simulink model "encoder_M_T"  (R2012b)
settings: Solver=ode45  StartTime=0.0  StopTime=10.0  RelTol=1e-3
libraries: simulink x4
settings Model: Creator=Juliano  LastModifiedBy=Juliano

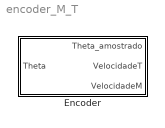
== system encoder_M_T ==
  Encoder : Subsystem  mask{Nr=500}
      mask prompts: Nr "Número de pulsos por revolução"

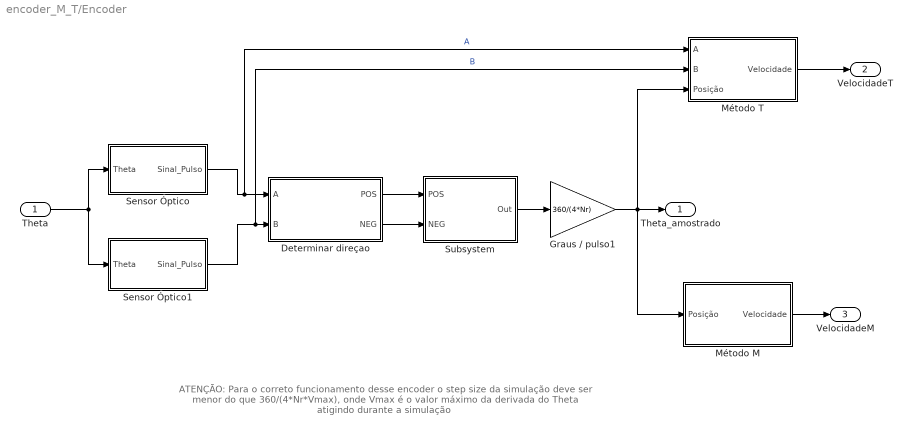
== system encoder_M_T/Encoder ==
  note: ATENÇÃO: Para o correto funcionamento desse encoder o step size da simulação deve ser menor do que 360/(4*Nr*Vmax),
      | onde Vmax é o valor máximo da derivada do Theta atigindo durante a simulação
  Theta : Inport
  Determinar direçao : Subsystem
  Graus / pulso1 : Gain  Gain=360/(4*Nr)  OutDataTypeStr=double
  Método M : Subsystem  mask{Ts=0.1}
      mask prompts: Ts "Sampling time"
  Método T : Subsystem  mask{m=10}
      mask prompts: m "Número de pulsos que o bloco espera para calcular a velocidade média"
  Sensor Óptico : Subsystem
  Sensor Óptico1 : Subsystem
  Subsystem : Subsystem
  Theta_amostrado : Outport
  VelocidadeT : Outport  Port=2
  VelocidadeM : Outport  Port=3
  wires:
  Método M/1(Velocidade) -> VelocidadeM/1
  Método T/1(Velocidade) -> VelocidadeT/1
  Theta/1 -> Sensor Óptico/1(Theta), Sensor Óptico1/1(Theta)
  Graus / pulso1/1 -> Theta_amostrado/1, Método T/3(Posição), Método M/1(Posição)
  Subsystem/1(Out) -> Graus / pulso1/1
  Determinar direçao/2(NEG) -> Subsystem/2(NEG)
  Determinar direçao/1(POS) -> Subsystem/1(POS)
  Sensor Óptico1/1(Sinal_Pulso) -> Determinar direçao/2(B), Método T/2(B)  "B"
  Sensor Óptico/1(Sinal_Pulso) -> Método T/1(A), Determinar direçao/1(A)  "A"

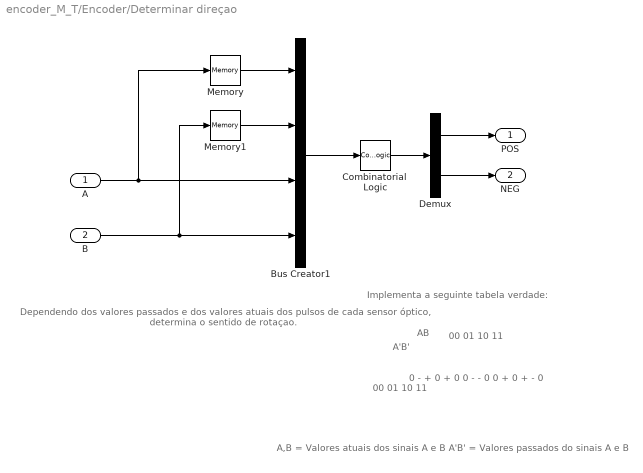
== system encoder_M_T/Encoder/Determinar direçao ==
  note: Dependendo dos valores passados e dos valores atuais
      | dos pulsos de cada sensor óptico, determina o sentido
      | de rotaçao.
  note: 00
      | 01
      | 10
      | 11
  note: 00 01 10 11
  note: 0	-	+	0
      | +	0	0	-
      | -	0	0	+
      | 0	+	-	0
  note: Implementa a seguinte tabela verdade:
  note: AB
  note: A'B'
  note: A,B = Valores atuais dos sinais A e B
      | A'B' = Valores passados do sinais A e B
  A : Inport
  B : Inport  Port=2
  Bus Creator1 : BusCreator
  Combinatorial  Logic : CombinatorialLogic  TruthTable=[ 0 0 ; 0 1 ; 1 0 ; 0 0 ; 1 0 ; 0 0 ; 0 0 ; 0 1 ; 0 1 ; 0 0 ; 0 0 ; 1 0 ; 0 0 ; 1 0 ; 0 1 ; 0 0]
  Demux : Demux  Outputs=2
  Memory : Memory
  Memory1 : Memory
  POS : Outport
  NEG : Outport  Port=2
  wires:
  B/1 -> Bus Creator1/4, Memory1/1
  Memory1/1 -> Bus Creator1/2
  Bus Creator1/1 -> Combinatorial  Logic/1
  Memory/1 -> Bus Creator1/1
  Combinatorial  Logic/1 -> Demux/1
  Demux/2 -> NEG/1
  A/1 -> Bus Creator1/3, Memory/1
  Demux/1 -> POS/1

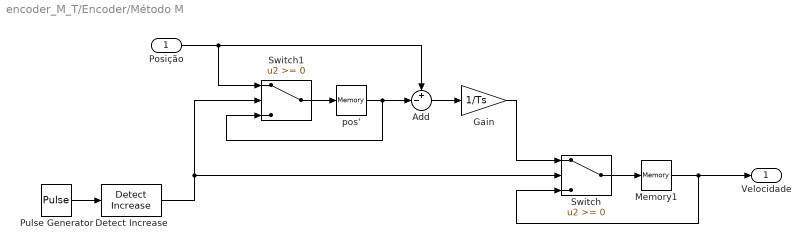
== system encoder_M_T/Encoder/Método M ==
  Posição : Inport
  Add : Sum  Inputs=+-|
  Detect Increase : simulink/Logic and Bit Operations/Detect Increase  vinit=0.0  InputProcessing=Inherited  OutDataTypeStr=boolean
  Gain : Gain  Gain=1/Ts
  Memory1 : Memory
  Pulse Generator : DiscretePulseGenerator  PulseType=Time based  Period=Ts  PulseWidth=50
  Switch : Switch
  Switch1 : Switch
  pos' : Memory
  Velocidade : Outport
  wires:
  Detect Increase/1 -> Switch1/2, Switch/2
  Gain/1 -> Switch/1
  Posição/1 -> Add/1, Switch1/1
  Memory1/1 -> Switch/3, Velocidade/1
  Switch/1 -> Memory1/1
  Switch1/1 -> pos'/1
  Add/1 -> Gain/1
  Pulse Generator/1 -> Detect Increase/1
  pos'/1 -> Switch1/3, Add/2

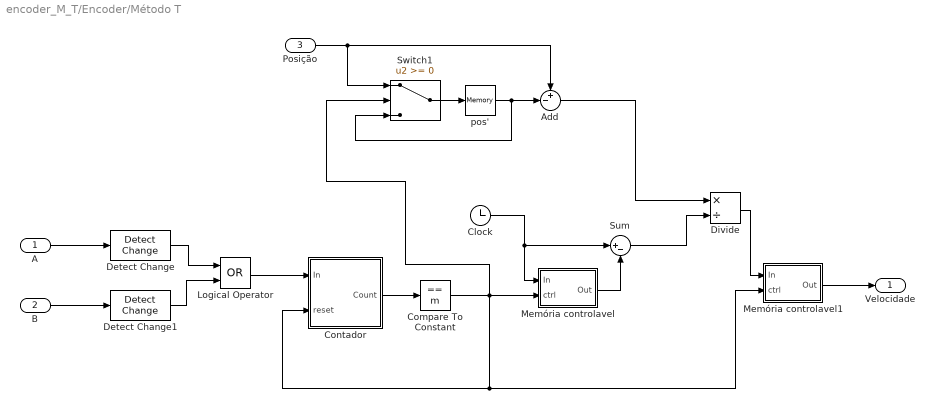
== system encoder_M_T/Encoder/Método T ==
  A : Inport
  B : Inport  Port=2
  Posição : Inport  Port=3
  Add : Sum  Inputs=+-|
  Clock : Clock
  Compare To Constant : simulink/Logic and Bit Operations/Compare To Constant  relop===  const=m  OutDataTypeStr=boolean
  Contador : Subsystem
  Detect Change : simulink/Logic and Bit Operations/Detect Change  vinit=0  InputProcessing=Inherited  OutDataTypeStr=boolean
  Detect Change1 : simulink/Logic and Bit Operations/Detect Change  vinit=0  InputProcessing=Inherited  OutDataTypeStr=boolean
  Divide : Product  Inputs=*/
  Logical Operator : Logic  Operator=OR  AllPortsSameDT=off  OutDataTypeStr=boolean
  Memória controlavel : Subsystem
  Memória controlavel1 : Subsystem
  Sum : Sum  Inputs=|+-
  Switch1 : Switch
  pos' : Memory
  Velocidade : Outport
  wires:
  Posição/1 -> Add/1, Switch1/1
  Switch1/1 -> pos'/1
  pos'/1 -> Switch1/3, Add/2
  Memória controlavel1/1(Out) -> Velocidade/1
  Compare To Constant/1 -> Memória controlavel/2(ctrl), Switch1/2, Contador/2(reset), Memória controlavel1/2(ctrl)
  Clock/1 -> Memória controlavel/1(In), Sum/1
  Add/1 -> Divide/1
  Sum/1 -> Divide/2
  Memória controlavel/1(Out) -> Sum/2
  Divide/1 -> Memória controlavel1/1(In)
  Contador/1(Count) -> Compare To Constant/1
  Logical Operator/1 -> Contador/1(In)
  Detect Change1/1 -> Logical Operator/2
  Detect Change/1 -> Logical Operator/1
  B/1 -> Detect Change1/1
  A/1 -> Detect Change/1

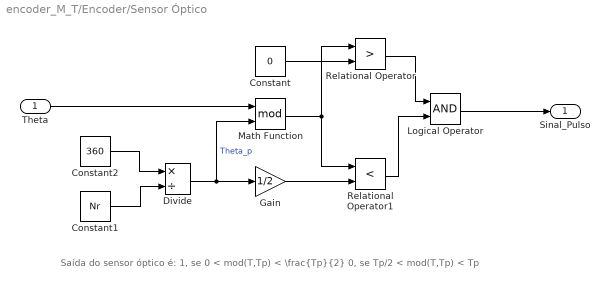
== system encoder_M_T/Encoder/Sensor Óptico ==
  note: Saída do sensor óptico é:
      | 1, se	0 < mod(T,Tp) < \frac{Tp}{2}
      |  0, se      Tp/2 < mod(T,Tp) < Tp
  Theta : Inport
  Constant : Constant  Value=0
  Constant1 : Constant  Value=Nr
  Constant2 : Constant  Value=360
  Divide : Product  Inputs=*/
  Gain : Gain  Gain=1/2
  Logical Operator : Logic  AllPortsSameDT=off  OutDataTypeStr=boolean
  Math Function : Math  Operator=mod  SaturateOnIntegerOverflow=on
  Relational Operator : RelationalOperator  Operator=>  OutDataTypeStr=boolean
  Relational Operator1 : RelationalOperator  Operator=<  OutDataTypeStr=boolean
  Sinal_Pulso : Outport
  wires:
  Constant1/1 -> Divide/2
  Constant2/1 -> Divide/1
  Logical Operator/1 -> Sinal_Pulso/1
  Gain/1 -> Relational Operator1/2
  Divide/1 -> Gain/1, Math Function/2  "Theta_p"
  Constant/1 -> Relational Operator/2
  Relational Operator1/1 -> Logical Operator/2
  Relational Operator/1 -> Logical Operator/1
  Theta/1 -> Math Function/1
  Math Function/1 -> Relational Operator/1, Relational Operator1/1

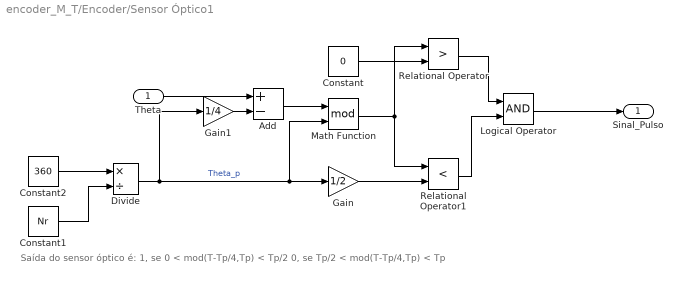
== system encoder_M_T/Encoder/Sensor Óptico1 ==
  note: Saída do sensor óptico é:
      | 1, se	0 < mod(T-Tp/4,Tp) < Tp/2
      |  0, se     Tp/2 < mod(T-Tp/4,Tp) < Tp
  Theta : Inport
  Add : Sum  Inputs=+-
  Constant : Constant  Value=0
  Constant1 : Constant  Value=Nr
  Constant2 : Constant  Value=360
  Divide : Product  Inputs=*/
  Gain : Gain  Gain=1/2
  Gain1 : Gain  Gain=1/4
  Logical Operator : Logic  AllPortsSameDT=off  OutDataTypeStr=boolean
  Math Function : Math  Operator=mod  SaturateOnIntegerOverflow=on
  Relational Operator : RelationalOperator  Operator=>  OutDataTypeStr=boolean
  Relational Operator1 : RelationalOperator  Operator=<  OutDataTypeStr=boolean
  Sinal_Pulso : Outport
  wires:
  Gain1/1 -> Add/2
  Theta/1 -> Add/1
  Add/1 -> Math Function/1
  Math Function/1 -> Relational Operator1/1, Relational Operator/1
  Relational Operator/1 -> Logical Operator/1
  Relational Operator1/1 -> Logical Operator/2
  Constant/1 -> Relational Operator/2
  Divide/1 -> Math Function/2, Gain/1, Gain1/1  "Theta_p"
  Gain/1 -> Relational Operator1/2
  Logical Operator/1 -> Sinal_Pulso/1
  Constant2/1 -> Divide/1
  Constant1/1 -> Divide/2

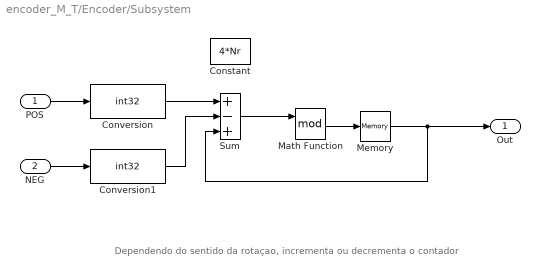
== system encoder_M_T/Encoder/Subsystem ==
  note: Dependendo do sentido da rotaçao, incrementa ou decrementa o contador
  POS : Inport
  NEG : Inport  Port=2
  Constant : Constant  Value=4*Nr
  Conversion : DataTypeConversion  OutDataTypeStr=int32
  Conversion1 : DataTypeConversion  OutDataTypeStr=int32
  Math Function : Math  Operator=mod  SaturateOnIntegerOverflow=on
  Memory : Memory
  Sum : Sum  Inputs=+-+
  Out : Outport
  wires:
  NEG/1 -> Conversion1/1
  Conversion1/1 -> Sum/2
  Conversion/1 -> Sum/1
  POS/1 -> Conversion/1
  Math Function/1 -> Memory/1
  Memory/1 -> Sum/3, Out/1
  Sum/1 -> Math Function/1

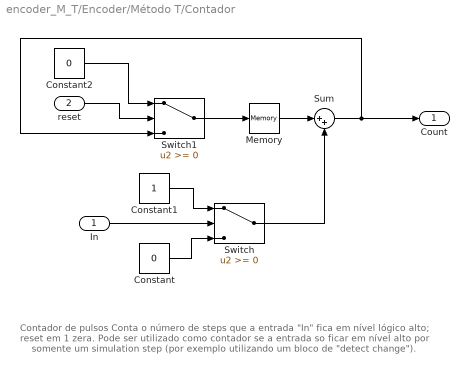
== system encoder_M_T/Encoder/Método T/Contador ==
  note: Contador de pulsos
      |
      | Conta o número de steps que a entrada "In" fica em nível lógico alto; reset em 1 zera.
      | Pode ser utilizado como contador se a entrada so ficar em nível alto por somente um
      | simulation step (por exemplo utilizando um bloco de "detect change").
  In : Inport
  reset : Inport  Port=2
  Constant : Constant  Value=0
  Constant1 : Constant
  Constant2 : Constant  Value=0
  Memory : Memory
  Sum : Sum  Inputs=|++
  Switch : Switch
  Switch1 : Switch
  Count : Outport
  wires:
  Constant/1 -> Switch/3
  Memory/1 -> Sum/1
  Constant1/1 -> Switch/1
  Sum/1 -> Switch1/3, Count/1
  Switch/1 -> Sum/2
  In/1 -> Switch/2
  reset/1 -> Switch1/2
  Constant2/1 -> Switch1/1
  Switch1/1 -> Memory/1

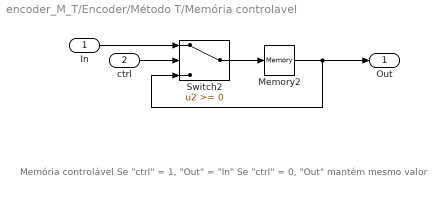
== system encoder_M_T/Encoder/Método T/Memória controlavel ==
  note: Memória controlável
      |
      | Se "ctrl" = 1, "Out" = "In"
      | Se "ctrl" = 0, "Out" mantém mesmo valor
  In : Inport
  ctrl : Inport  Port=2
  Memory2 : Memory
  Switch2 : Switch
  Out : Outport
  wires:
  In/1 -> Switch2/1
  ctrl/1 -> Switch2/2
  Memory2/1 -> Switch2/3, Out/1
  Switch2/1 -> Memory2/1

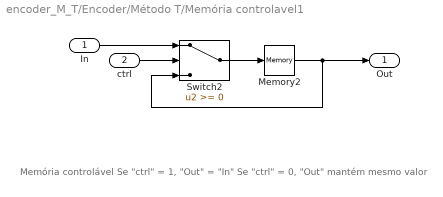
== system encoder_M_T/Encoder/Método T/Memória controlavel1 ==
  note: Memória controlável
      |
      | Se "ctrl" = 1, "Out" = "In"
      | Se "ctrl" = 0, "Out" mantém mesmo valor
  In : Inport
  ctrl : Inport  Port=2
  Memory2 : Memory
  Switch2 : Switch
  Out : Outport
  wires:
  Switch2/1 -> Memory2/1
  Memory2/1 -> Out/1, Switch2/3
  ctrl/1 -> Switch2/2
  In/1 -> Switch2/1
